simulink model "Ej_3_1_m1"  (R2022b)
settings: Solver=VariableStepAuto  StartTime=0.0  StopTime=10.0  RelTol=1e-3
settings Model: Creator=rrilo  LastModifiedBy=rrilo

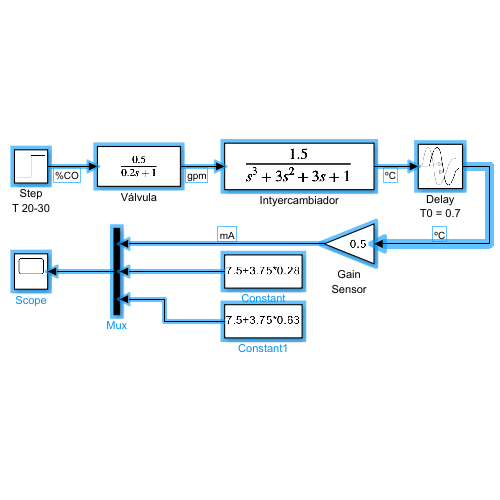
[thumbnail: Simulink's stored preview of the top-level diagram]
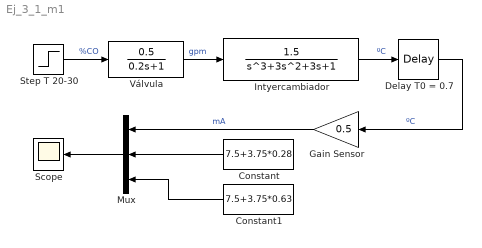
== system Ej_3_1_m1 ==
  Constant : Constant  Value=7.5+3.75*0.28
  Constant1 : Constant  Value=7.5+3.75*0.63
  Delay T0 = 0.7 : TransportDelay  DelayTime=0.7
  Gain Sensor : Gain  Gain=0.5
  Intyercambiador : TransferFcn  Numerator=[1.5]  Denominator=[1 3 3 1]
  Mux : Mux  Inputs=3
  Scope : Scope
  Step T 20-30 : Step  Time=20  Before=20  After=30  SampleTime=0
  Válvula : TransferFcn  Numerator=[0.5]  Denominator=[0.2 1]
  wires:
  Gain Sensor/1 -> Mux/1  "mA"
  Constant1/1 -> Mux/3
  Constant/1 -> Mux/2
  Intyercambiador/1 -> Delay T0 = 0.7/1  "ºC"
  Step T 20-30/1 -> Válvula/1  "%CO"
  Mux/1 -> Scope/1
  Válvula/1 -> Intyercambiador/1  "gpm"
  Delay T0 = 0.7/1 -> Gain Sensor/1  "ºC"
